simulink model "clik_transpose"  (Simulink 10.2)
settings: Solver=VariableStepAuto  StartTime=0.0  StopTime=4  RelTol=1e-3
undefined symbols (not defined in the file or in its folder): DiscIntNeverNeededParam, q0, Tc
settings Model: Creator=sujay  LastModifiedBy=Megha
settings DataIOCC: SaveFormat=Dataset  SignalLoggingSaveFormat=Dataset  ReturnWorkspaceOutputs=on
settings OptimizationCC: LifeSpan=auto
settings DebuggingCC: UnderspecifiedInitializationDetection=Simplified  MergeDetectMultiDrivingBlocksExec=error  FcnCallInpInsideContextMsg=error  SFUnexpectedBacktrackingDiag=error  SFNoUnconditionalDefaultTransitionDiag=error  SFExecutionAtInitializationDiag=warning
settings HardwareCC: ProdBitPerPointer=64  ProdBitPerSizeT=64  ProdBitPerPtrDiffT=64  ProdLargestAtomicFloat=Float  ProdIntDivRoundTo=Zero  ProdEndianess=LittleEndian  ProdWordSize=64  ProdHWDeviceType=Intel->x86-64 (Windows64)
settings ModelReferenceCC: PropagateSignalLabelsOutOfModel=on
settings SFSimCC: SimUseLocalCustomCode=on
settings RTWCC: RTWUseLocalCustomCode=on
settings CodeAppCC: StateflowObjectComments=off
settings GRTTargetCC: TargetLangStandard=C99 (ISO)  CombineOutputUpdateFcns=on  GRTInterface=off
settings ConfigComp: CovMetricSettings=dwe  CovSaveCumulativeToWorkspaceVar=off  CovSaveSingleToWorkspaceVar=off  CovExternalEMLEnable=on

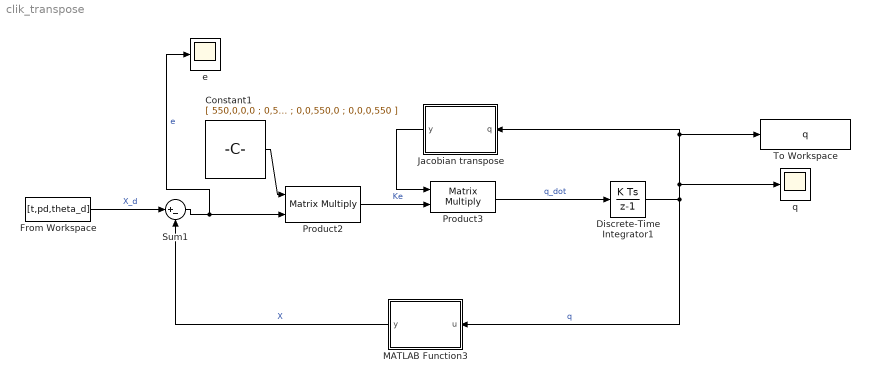
== system clik_transpose ==
  Constant1 : Constant  Value=[ 550,0,0,0 ; 0,550,0,0 ; 0,0,550,0 ; 0,0,0,550 ]  VectorParams1D=off
  Discrete-Time Integrator1 : DiscreteIntegrator  InitialCondition=q0  SampleTime=Tc  ICPrevOutput=DiscIntNeverNeededParam  ICPrevScaledInput=DiscIntNeverNeededParam
  From Workspace : FromWorkspace  VariableName=[t,pd,theta_d]
  Jacobian transpose : MATLAB Function  TreatAsAtomicUnit=on
  MATLAB Function3 : MATLAB Function  TreatAsAtomicUnit=on
  Product2 : Product  Multiplication=Matrix(*)
  Product3 : Product  Multiplication=Matrix(*)
  Sum1 : Sum  Inputs=|+-
  To Workspace : ToWorkspace  VariableName=q  SampleTime=-1
  e : Scope
  q : Scope
  wires:
  Product3/1 -> Discrete-Time Integrator1/1  "q_dot"
  MATLAB Function3/1(y) -> Sum1/2  "X"
  Product2/1 -> Product3/2  "Ke"
  Discrete-Time Integrator1/1 -> Jacobian transpose/1(q), To Workspace/1, q/1, MATLAB Function3/1(u)  "q"
  Constant1/1 -> Product2/1
  Sum1/1 -> e/1, Product2/2  "e"
  Jacobian transpose/1(y) -> Product3/1
  From Workspace/1 -> Sum1/1  "X_d"

== matlab function Jacobian transpose ==
  data: q input double; y output double
function y = Jacobian(q)

J_transpose = transpose(Jacobian(q));

y = J_transpose;

== matlab function MATLAB Function3 ==
  data: u input double; y output double
function y = Kinematics(u)

y = [ 0.5*(cos(u(1,1)+u(2,1))+cos(u(1,1))) ; 0.5*(sin(u(1,1)+u(2,1))+sin(u(1,1))) ; (1 - u(3,1)) ; u(1,1)+u(2,1)+u(4,1) ];

end
